simulink model "Competition_Motor_Control_Model"  (R2017b)
settings: Solver=FixedStepDiscrete  StartTime=0.0  StopTime=inf  FixedStep=0.02  RelTol=1e-3  EnableMultiTasking=on
InitFcn:
  | Step_Size=0.02;
  | Speed_Steering_Right_Tire = [0 0 0.5 1 1 0.8 0.3 0 0];
  | Speed_Steering_Left_Tire=Speed_Steering_Right_Tire(end:-1:1);
  | Speed_Steering_Speed_Vector=4.*[-16 -15 -10 -5 0 5 10 15 16 ];
  | %plot(Speed_Steering_Speed_Vector,Speed_Steering_Right_Tire,'b',Speed_Steering_Speed_Vector,Speed_Steering_Left_Tire,'r');
  | 
  | Steering_Dead_Zone = 5;
libraries: frdmtfcshieldlib x10, Autonomous_Vehicle_Competition x2, nxpcupcompanionlib_R2016b x1, frdmkl25zlib x1
settings Model: SimulationMode=external  ExtModeTrigDuration=1  Creator=Lalla  LastModifiedBy=daren
settings SolverCC: AutoInsertRateTranBlk=on
settings DataIOCC: LimitDataPoints=on  SaveFormat=Array
settings OptimizationCC: LifeSpan=1  MaxStackSize=64
settings DebuggingCC: SolverPrmCheckMsg=warning  MultiTaskCondExecSysMsg=none  UnconnectedInputMsg=error  UnconnectedOutputMsg=error  UnconnectedLineMsg=error  AllowSymbolicDim=off  SFUnexpectedBacktrackingDiag=warning  SFNoUnconditionalDefaultTransitionDiag=warning  SFExecutionAtInitializationDiag=none
settings HardwareCC: ProdBitPerPointer=32  ProdBitPerSizeT=32  ProdBitPerPtrDiffT=32  ProdLargestAtomicInteger=Long  ProdLargestAtomicFloat=Double  ProdIntDivRoundTo=Undefined  ProdWordSize=32  ProdHWDeviceType=ARM Compatible->ARM Cortex
settings ModelReferenceCC: PropagateSignalLabelsOutOfModel=off
settings SFSimCC: MATLABDynamicMemAlloc=off
settings RTWCC: SystemTargetFile=ert.tlc  HardwareBoard=NXP FRDM-KL25Z  TLCOptions=-aInlineSetEventsForThisBaseRateFcn=TLC_FALSE -aSuppressMultiTaskScheduler=TLC_FALSE -aRateBasedStepFcn=1  TemplateMakefile=ert_default_tmf  Toolchain=GNU Tools for ARM Embedded Processors  BuildConfiguration=Faster Runs
settings CodeAppCC: IgnoreCustomStorageClasses=off  StateflowObjectComments=on
settings ERTTargetCC: MultiwordLength=2048  SupportNonInlinedSFcns=on  SupportVariableSizeSignals=on  ExtModeTransport=1  ExtModeMexFile=ext_serial_win32_comm  ExtModeMexArgs=0 11  ConvertIfToSwitch=off  SuppressUnreachableDefaultCases=off
settings ConfigComp: CovMetricSettings=dw  CovHtmlReporting=on  CovSaveCumulativeToWorkspaceVar=on  CovSaveSingleToWorkspaceVar=on  CovExternalEMLEnable=off  CovSFcnEnable=off

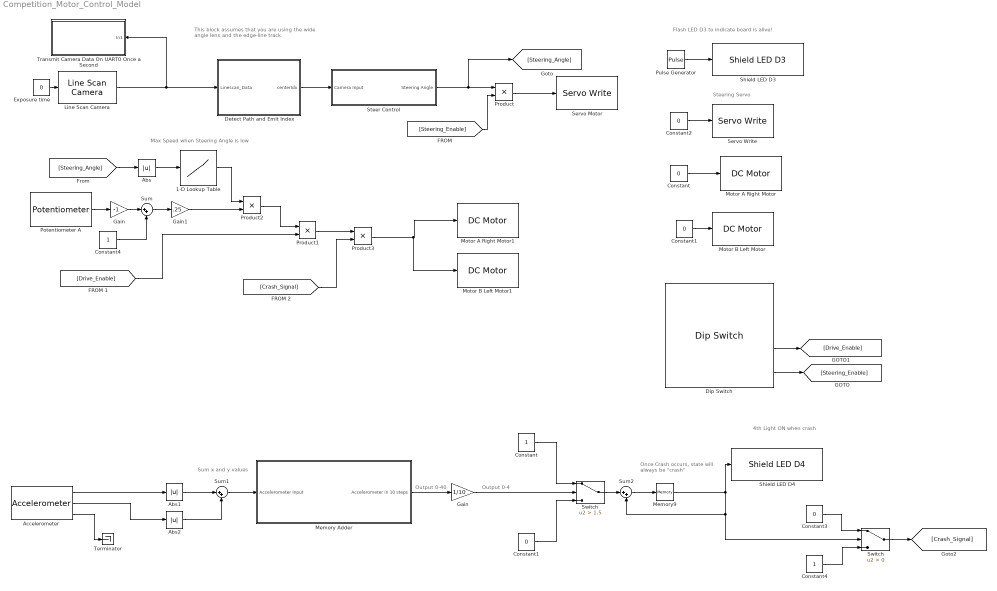
== system Competition_Motor_Control_Model ==
  note: Max Speed when Steering Angle is low
  note: Once Crash occurs, state will always be "crash"
  note: Sum x and y values
  note: Output 0-40
  note: This block assumes that you are using the wide angle lens
      | and the edge-line track.
  note: Steering Servo
  note: Flash LED D3 to indicate board is alive!
  note: Output 0-4
  note: 4th Light ON when crash
  "1-D Lookup Table " : Lookup_n-D  NumberOfTableDimensions=1  BreakpointsForDimension1=[0 10 30]  Table=[1 1 0.5]  ExtrapMethod=Clip  UseLastTableValue=on  InternalRulePriority=Speed  RndMeth=Simplest  InputSameDT=on
  Abs : Abs
  "Abs1 " : Abs
  "Abs2 " : Abs
  Accelerometer : nxpcupcompanionlib_R2016b/Accelerometer  SampleTime=-1
      settings: SourceProductName=NXP Cup Companion
  Constant : Constant  Value=0
  "Constant " : Constant
  Constant1 : Constant  Value=0
  "Constant1 " : Constant  Value=0
  Constant2 : Constant  Value=0
  "Constant3 " : Constant  Value=0
  Constant4 : Constant
  "Constant4 " : Constant
  Detect Path and Emit Index : MATLAB Function  TreatAsAtomicUnit=on
  Dip Switch : frdmtfcshieldlib/Dip Switch  SampleTime=-1
      settings: SourceProductName=Simulink Coder Support Package for NXP FRDM-KL25Z Board  SourceProductBaseCode=EC_FREEDOM_BOARD
  Exposure time : Constant  Value=0
  Gain : Gain  Gain=-1
  "Gain " : Gain  Gain=1/10
  Gain1 : Gain  Gain=.25
  Line Scan Camera : frdmtfcshieldlib/Line Scan Camera  CameraHeader=0  SampleTime=.02
      settings: SourceProductName=Simulink Coder Support Package for NXP FRDM-KL25Z Board  SourceProductBaseCode=EC_FREEDOM_BOARD
  Memory Adder : Subsystem
  "Memory9 " : Memory
  Motor A Right Motor : frdmtfcshieldlib/DC Motor  WhichMotor=A
      settings: SourceProductName=Simulink Coder Support Package for NXP FRDM-KL25Z Board  SourceProductBaseCode=EC_FREEDOM_BOARD
  Motor A Right Motor1 : frdmtfcshieldlib/DC Motor  WhichMotor=A
      settings: SourceProductName=Simulink Coder Support Package for NXP FRDM-KL25Z Board  SourceProductBaseCode=EC_FREEDOM_BOARD
  Motor B Left Motor : frdmtfcshieldlib/DC Motor  WhichMotor=B
      settings: SourceProductName=Simulink Coder Support Package for NXP FRDM-KL25Z Board  SourceProductBaseCode=EC_FREEDOM_BOARD
  Motor B Left Motor1 : frdmtfcshieldlib/DC Motor  WhichMotor=B
      settings: SourceProductName=Simulink Coder Support Package for NXP FRDM-KL25Z Board  SourceProductBaseCode=EC_FREEDOM_BOARD
  Potentiometer A : frdmtfcshieldlib/Potentiometer  WhichPot=A  SampleTime=-1
      settings: SourceProductName=Simulink Coder Support Package for NXP FRDM-KL25Z Board  SourceProductBaseCode=EC_FREEDOM_BOARD
  Product{,1..3} (4 alike) : Product
  Pulse Generator : DiscretePulseGenerator  PulseType=Time based  Period=1  PulseWidth=50
  "Servo Motor " : frdmtfcshieldlib/Servo Write  WhichServo=0  minAngle=-90  maxAngle=90
      settings: SourceProductName=Simulink Coder Support Package for NXP FRDM-KL25Z Board  SourceProductBaseCode=EC_FREEDOM_BOARD
  Servo Write : frdmtfcshieldlib/Servo Write  WhichServo=0  minAngle=-90  maxAngle=90
      settings: SourceProductName=Simulink Coder Support Package for NXP FRDM-KL25Z Board  SourceProductBaseCode=EC_FREEDOM_BOARD
  Shield LED D3 : Autonomous_Vehicle_Competition/Shield LED D3
      settings: SourceProductName=Autonomous Vehicle Competition
  "Shield LED D4 " : Autonomous_Vehicle_Competition/Shield LED D4
      settings: SourceProductName=Autonomous Vehicle Competition
  Steer Control : Subsystem
  Sum : Sum  Inputs=|++
  Sum1 : Sum  Inputs=|++
  Sum2 : Sum  Inputs=|++
  Switch : Switch  Criteria=u2 > Threshold
  "Switch " : Switch  Criteria=u2 > Threshold  Threshold=1.5
  "Terminator " : Terminator
  Transmit Camera Data On UART0 Once a Second : Subsystem  TreatAsAtomicUnit=on  SystemSampleTime=.26
  wires:
  Pulse Generator/1 -> Shield LED D3/1
  Exposure time/1 -> Line Scan Camera/1
  Line Scan Camera/1 -> Transmit Camera Data On UART0 Once a Second/1(In1), Detect Path and Emit Index/1(Linescan_Data)
  Constant/1 -> Motor A Right Motor/1
  Constant1/1 -> Motor B Left Motor/1
  Constant2/1 -> Servo Write/1
  Product/1 -> "Servo Motor "/1
  Dip Switch/4 -> [Steering_Enable]
  [Steering_Enable] -> Product/2
  Detect Path and Emit Index/1(centerIdx) -> Steer Control/1(Camera Input)
  Steer Control/1(Steering Angle) -> [Steering_Angle], Product/1
  Dip Switch/3 -> [Drive_Enable]
  [Drive_Enable] -> Product1/2
  Potentiometer A/1 -> Gain/1
  Gain/1 -> Sum/1
  Constant4/1 -> Sum/2
  Sum/1 -> Gain1/1
  Gain1/1 -> Product2/2
  [Steering_Angle] -> Abs/1
  Abs/1 -> "1-D Lookup Table "/1
  "1-D Lookup Table "/1 -> Product2/1
  Product2/1 -> Product1/1
  Switch/1 -> [Crash_Signal]
  "Constant "/1 -> "Switch "/1
  "Constant1 "/1 -> "Switch "/3
  "Constant3 "/1 -> Switch/1
  Accelerometer/2 -> "Abs2 "/1
  Accelerometer/3 -> "Terminator "/1
  "Memory9 "/1 -> Switch/2, Sum2/2, "Shield LED D4 "/1
  "Abs2 "/1 -> Sum1/2
  Sum2/1 -> "Memory9 "/1
  "Constant4 "/1 -> Switch/3
  "Abs1 "/1 -> Sum1/1
  "Switch "/1 -> Sum2/1
  "Gain "/1 -> "Switch "/2
  Accelerometer/1 -> "Abs1 "/1
  Sum1/1 -> Memory Adder/1(Accelerometer Input)
  Memory Adder/1(Accelerometer in 10 steps) -> "Gain "/1
  Product3/1 -> Motor B Left Motor1/1, Motor A Right Motor1/1
  Product1/1 -> Product3/1
  [Crash_Signal] -> Product3/2

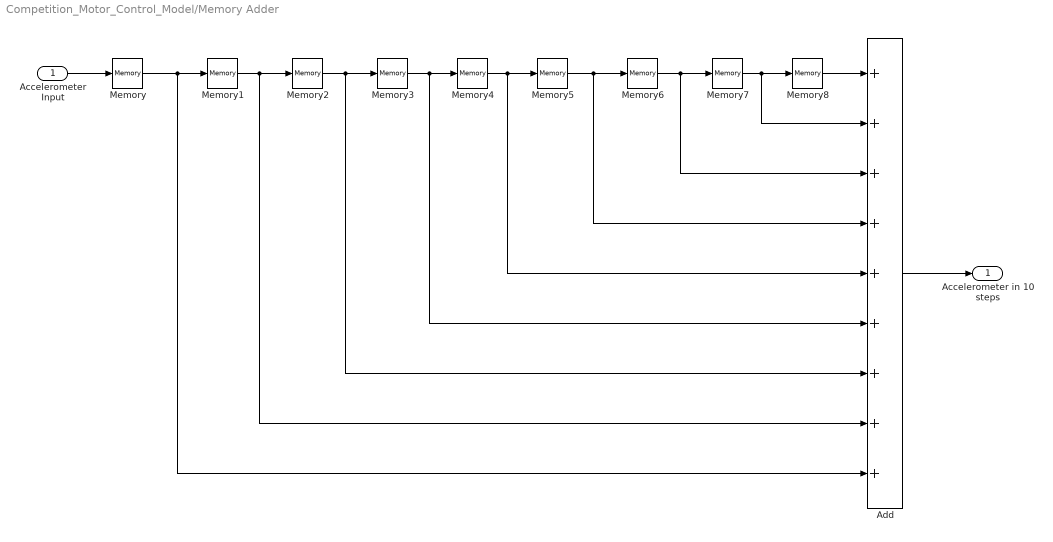
== system Competition_Motor_Control_Model/Memory Adder ==
  Accelerometer Input : Inport
  Add : Sum  Inputs=+++++++++
  "Memory " : Memory
  "Memory1 " : Memory
  "Memory2 " : Memory
  "Memory3 " : Memory
  "Memory4 " : Memory
  "Memory5 " : Memory
  "Memory6 " : Memory
  "Memory7 " : Memory
  "Memory8 " : Memory
  Accelerometer in 10 steps : Outport
  wires:
  "Memory5 "/1 -> Add/4, "Memory6 "/1
  "Memory2 "/1 -> Add/7, "Memory3 "/1
  "Memory6 "/1 -> Add/3, "Memory7 "/1
  "Memory "/1 -> Add/9, "Memory1 "/1
  Accelerometer Input/1 -> "Memory "/1
  "Memory4 "/1 -> Add/5, "Memory5 "/1
  "Memory1 "/1 -> Add/8, "Memory2 "/1
  "Memory7 "/1 -> Add/2, "Memory8 "/1
  "Memory3 "/1 -> Add/6, "Memory4 "/1
  Add/1 -> Accelerometer in 10 steps/1
  "Memory8 "/1 -> Add/1

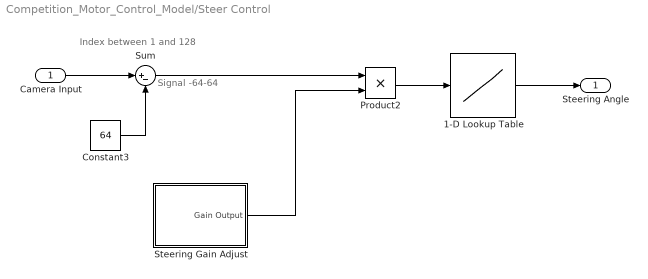
== system Competition_Motor_Control_Model/Steer Control ==
  note: Signal -64-64
  note: Index between 1 and 128
  Camera Input : Inport
  "1-D Lookup Table " : Lookup_n-D  NumberOfTableDimensions=1  BreakpointsForDimension1=[-30 -2 2 30]  Table=[-30 0 0 30]  ExtrapMethod=Clip  UseLastTableValue=on  InternalRulePriority=Speed  RndMeth=Simplest  InputSameDT=on
  Constant3 : Constant  Value=64
  Product2 : Product
  Steering Gain Adjust : Subsystem
  Sum : Sum  Inputs=|+-
  Steering Angle : Outport
  wires:
  Steering Gain Adjust/1(Gain Output) -> Product2/2
  Camera Input/1 -> Sum/1
  Product2/1 -> "1-D Lookup Table "/1
  Sum/1 -> Product2/1
  Constant3/1 -> Sum/2
  "1-D Lookup Table "/1 -> Steering Angle/1

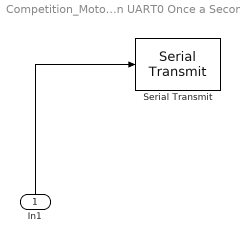
== system Competition_Motor_Control_Model/Transmit Camera Data On UART0 Once a Second ==
  In1 : Inport
  Serial Transmit : frdmkl25zlib/Serial Transmit  uart=UART0  sendmode=printf
      settings: SourceProductName=Simulink Coder Support Package for NXP FRDM-KL25Z Board  SourceProductBaseCode=EC_FREEDOM_BOARD
  wires:
  In1/1 -> Serial Transmit/1

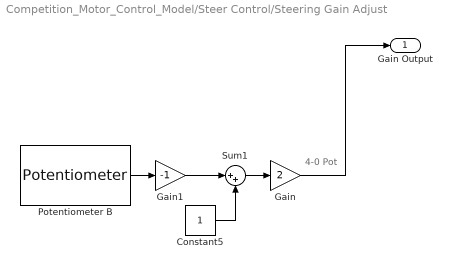
== system Competition_Motor_Control_Model/Steer Control/Steering Gain Adjust ==
  note: 4-0 Pot
  Constant5 : Constant
  Gain : Gain  Gain=2
  Gain1 : Gain  Gain=-1
  "Potentiometer B " : frdmtfcshieldlib/Potentiometer  WhichPot=B  SampleTime=-1
      settings: SourceProductName=Simulink Coder Support Package for NXP FRDM-KL25Z Board  SourceProductBaseCode=EC_FREEDOM_BOARD
  Sum1 : Sum  Inputs=|++
  Gain Output : Outport
  wires:
  Constant5/1 -> Sum1/2
  Gain1/1 -> Sum1/1
  "Potentiometer B "/1 -> Gain1/1
  Sum1/1 -> Gain/1
  Gain/1 -> Gain Output/1

== matlab function Competition_Motor_Control_Model/Detect Path and Emit Index ==
  data: centerIdx output single; Linescan_Data input
function centerIdx = CenterIdx(Linescan_Data)
% function centerIdx = CenterIdx(Linescan_Data)
% This function finds the current position of the track's
% center. 

%%---------------------------------------------------------------------------------------------
% The lines below are also inside  file "Full_High_School_Model_0_View_Camera.m"
% This m-file will display the camera data and also the edges and center of
% the track using the same algorithm the vehicle uses. If you modify the
% lines below, you must also modify the same lines in file
% "Full_High_School_Model_0_View_Camera.m".
% 

First_Edge=single(1);
Second_Edge=single(128);

% Calculate the threshold as 75% of the mean value of the bright section of
% the track.
Threshold=0.75*mean(Linescan_Data(40:80));

%Find the First Edge
for i=64:-1:2
    if Linescan_Data(i)<Threshold;
        First_Edge=single(i);
        break;
    end
end

% Find the Second Edge
for i=64:1:127
    if Linescan_Data(i)<Threshold;
        Second_Edge=single(i);
        break;
    end
end

% If the edge indices are valid, then calculate the 
% center as the average of the two edge indices.
if First_Edge>1 && Second_Edge<128
    centerIdx=(Second_Edge+First_Edge)/2;
else
    centerIdx=single(255);
end

%Paste changes to the lines above in inside  file "Full_High_School_Model_0_View_Camera.m"
%----------------------------------------------------------------------------------------------------------


%%end  minimum finding algorithm

end
